simulink model "DynTaskCon"  (Simulink 7.6)
settings: Solver=ode45  StartTime=0.0  StopTime=10.0  RelTol=1e-3
InitFcn:
  | eval('Config')
values from neighbouring files (symbols this model uses):
  a2 = 0    [Config.m]    (also in CtrPlatformCfg.m)
  a3 = 0    [Config.m]    (also in CtrPlatformCfg.m)
  a4 = 0    [Config.m]    (also in CtrPlatformCfg.m)
  a5 = 90    [Config.m]    (also in CtrPlatformCfg.m)
  a6 = 0    [Config.m]    (also in CtrPlatformCfg.m)
  Cen = Cen(:)'    [Config.m]    (also in CtrPlatformCfg.m; DynEulerTest.m = Cen'; EfDynCAD.m = [cen1,cen2,cen3,cen4,cen5,cen6]')
  freq = tvel/radius    (= 1)    [Config.m]    (also in CtrPlatformCfg.m)
  Ie1 = in1(:)'    [Config.m]    (also in CtrPlatformCfg.m; DynEulerTest.m = in1(:); EfDynCAD.m = in1(:))
  Ie2 = in2(:)'    [Config.m]    (also in CtrPlatformCfg.m; DynEulerTest.m = in2(:); EfDynCAD.m = in2(:))
  Ie3 = in3(:)'    [Config.m]    (also in CtrPlatformCfg.m; DynEulerTest.m = in3(:); EfDynCAD.m = in3(:))
  Ie4 = in4(:)'    [Config.m]    (also in CtrPlatformCfg.m; DynEulerTest.m = in4(:); EfDynCAD.m = in4(:))
  Ie5 = in5(:)'    [Config.m]    (also in CtrPlatformCfg.m; DynEulerTest.m = in5(:); EfDynCAD.m = in5(:))
  Ie6 = in6(:)'    [Config.m]    (also in CtrPlatformCfg.m; DynEulerTest.m = in6(:); EfDynCAD.m = in6(:))
  init_Endx = gd_init(1,4)    [Config.m]    (also in CtrPlatformCfg.m)
  init_Endy = gd_init(2,4)    [Config.m]    (also in CtrPlatformCfg.m)
  init_Endz = gd_init(3,4)    [Config.m]    (also in CtrPlatformCfg.m)
  init_Rot = gd_init(1:3,1:3)    [Config.m]    (also in CtrPlatformCfg.m)
  L = [l1 l2 l3 l4 l5 l6 l7 l8 l9]    [Config.m]    (also in CtrPlatformCfg.m)
  Ma = [ma1 ma2 ma3 ma4 ma5 ma6]    [Config.m]    (also in CtrPlatformCfg.m; DynEulerTest.m = [ma1; ma2; ma3; ma4; ma5; ma6]; EfDynCAD.m = [ma1 ma2 ma3 ma4 ma5 ma6]')
  tvel = 120    [Config.m]    (also in CtrPlatformCfg.m)
undefined symbols (not defined in the file or in its folder): a1
libraries: mblibv1 x35, simulink x9
(part 1 of 2)
settings Model: Creator=DAI Dan  LastModifiedBy=DAI Dan
settings SimMechanicsCC: VisOnUpdateDiagram=on  VisDuringSimulation=on

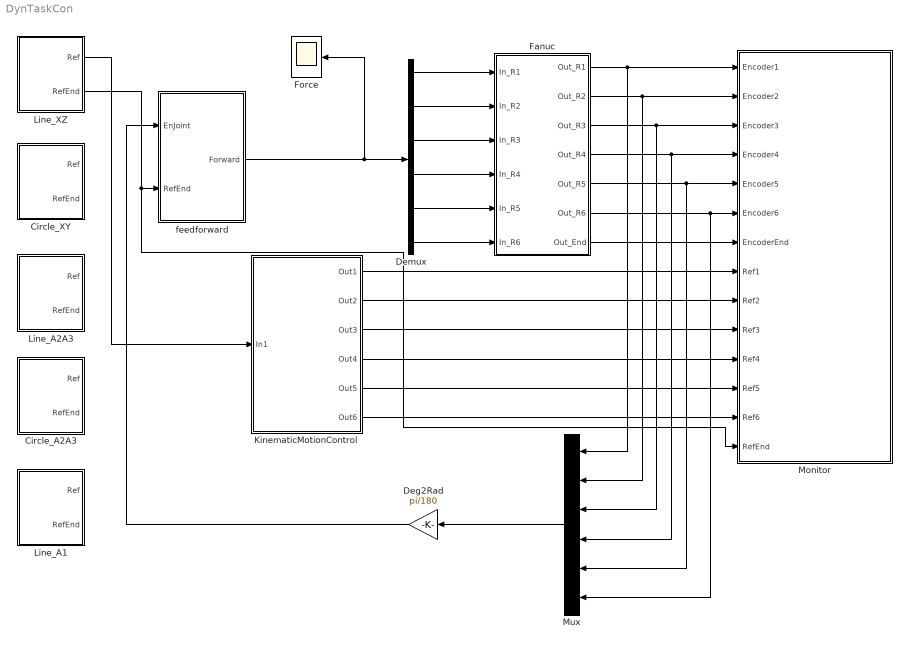
== system DynTaskCon ==
  Circle_A2A3 : Subsystem
  Circle_XY : Subsystem
  Deg2Rad : Gain  Gain=pi/180
  Demux : Demux  Outputs=6
  Fanuc : Subsystem
  Force : Scope
      settings: TimeRange=10  SaveName=ScopeData27
  KinematicMotionControl : Subsystem
  Line_A1 : Subsystem
  Line_A2A3 : Subsystem
  Line_XZ : Subsystem
  Monitor : Subsystem
  Mux : Mux  Inputs=6
  feedforward : Subsystem
  wires:
  Fanuc/1(Out_R1) -> Monitor/1(Encoder1), Mux/1
  Fanuc/2(Out_R2) -> Monitor/2(Encoder2), Mux/2
  Fanuc/3(Out_R3) -> Monitor/3(Encoder3), Mux/3
  Fanuc/4(Out_R4) -> Monitor/4(Encoder4), Mux/4
  Fanuc/5(Out_R5) -> Monitor/5(Encoder5), Mux/5
  Fanuc/6(Out_R6) -> Monitor/6(Encoder6), Mux/6
  Fanuc/7(Out_End) -> Monitor/7(EncoderEnd)
  KinematicMotionControl/1(Out1) -> Monitor/8(Ref1)
  KinematicMotionControl/2(Out2) -> Monitor/9(Ref2)
  KinematicMotionControl/3(Out3) -> Monitor/10(Ref3)
  KinematicMotionControl/4(Out4) -> Monitor/11(Ref4)
  KinematicMotionControl/5(Out5) -> Monitor/12(Ref5)
  KinematicMotionControl/6(Out6) -> Monitor/13(Ref6)
  Demux/1 -> Fanuc/1(In_R1)
  Demux/2 -> Fanuc/2(In_R2)
  Demux/3 -> Fanuc/3(In_R3)
  Demux/4 -> Fanuc/4(In_R4)
  Demux/5 -> Fanuc/5(In_R5)
  Demux/6 -> Fanuc/6(In_R6)
  Mux/1 -> Deg2Rad/1
  feedforward/1(Forward) -> Force/1, Demux/1
  Deg2Rad/1 -> feedforward/1(EnJoint)
  Line_XZ/1(Ref) -> KinematicMotionControl/1(In1)
  Line_XZ/2(RefEnd) -> Monitor/14(RefEnd), feedforward/2(RefEnd)

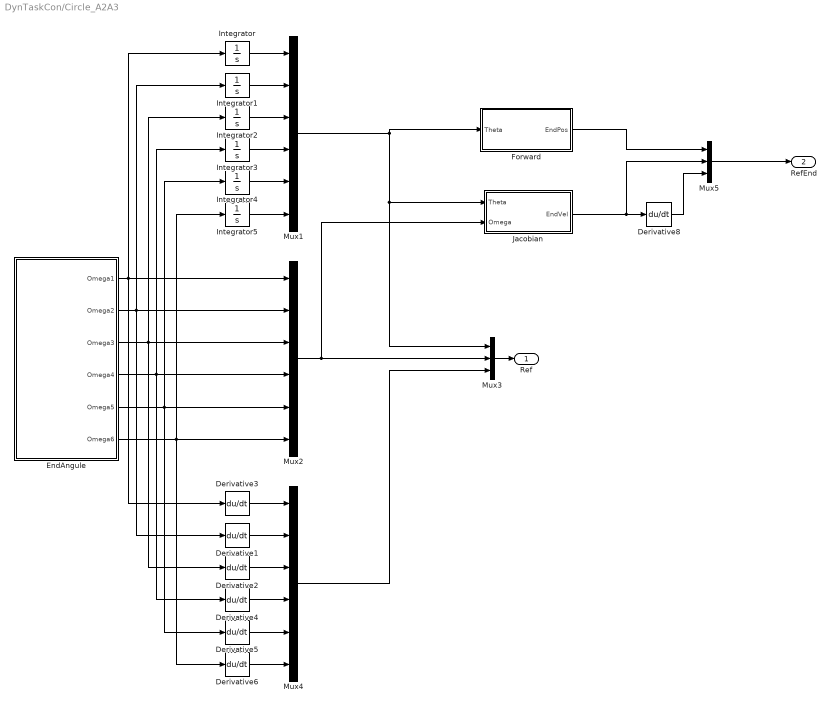
== system DynTaskCon/Circle_A2A3 ==
  Derivative{1..6,8} (7 alike) : Derivative
  EndAngule : Subsystem
  Forward : Stateflow chart  TreatAsAtomicUnit=on
  Integrator : Integrator  InitialCondition=a1/180*pi
  Integrator1 : Integrator  InitialCondition=a2/180*pi
  Integrator2 : Integrator  InitialCondition=a3/180*pi
  Integrator3 : Integrator  InitialCondition=a4/180*pi
  Integrator4 : Integrator  InitialCondition=a5/180*pi
  Integrator5 : Integrator  InitialCondition=a6/180*pi
  Jacobian : Stateflow chart  TreatAsAtomicUnit=on
  Mux1 : Mux  Inputs=6
  Mux2 : Mux  Inputs=6
  Mux3 : Mux  Inputs=3
  Mux4 : Mux  Inputs=6
  Mux5 : Mux  Inputs=3
  Ref : Outport
  RefEnd : Outport  Port=2
  wires:
  Mux3/1 -> Ref/1
  EndAngule/1(Omega1) -> Integrator/1, Mux2/1, Derivative3/1
  EndAngule/2(Omega2) -> Integrator1/1, Mux2/2, Derivative1/1
  EndAngule/3(Omega3) -> Integrator2/1, Mux2/3, Derivative2/1
  EndAngule/4(Omega4) -> Integrator3/1, Mux2/4, Derivative4/1
  EndAngule/5(Omega5) -> Integrator4/1, Mux2/5, Derivative5/1
  EndAngule/6(Omega6) -> Integrator5/1, Mux2/6, Derivative6/1
  Integrator/1 -> Mux1/1
  Integrator1/1 -> Mux1/2
  Integrator2/1 -> Mux1/3
  Integrator3/1 -> Mux1/4
  Integrator4/1 -> Mux1/5
  Integrator5/1 -> Mux1/6
  Derivative3/1 -> Mux4/1
  Derivative1/1 -> Mux4/2
  Derivative2/1 -> Mux4/3
  Derivative4/1 -> Mux4/4
  Derivative5/1 -> Mux4/5
  Derivative6/1 -> Mux4/6
  Mux2/1 -> Mux3/2, Jacobian/2(Omega)
  Mux1/1 -> Forward/1(Theta), Mux3/1, Jacobian/1(Theta)
  Mux4/1 -> Mux3/3
  Mux5/1 -> RefEnd/1
  Forward/1(EndPos) -> Mux5/1
  Jacobian/1(EndVel) -> Mux5/2, Derivative8/1
  Derivative8/1 -> Mux5/3

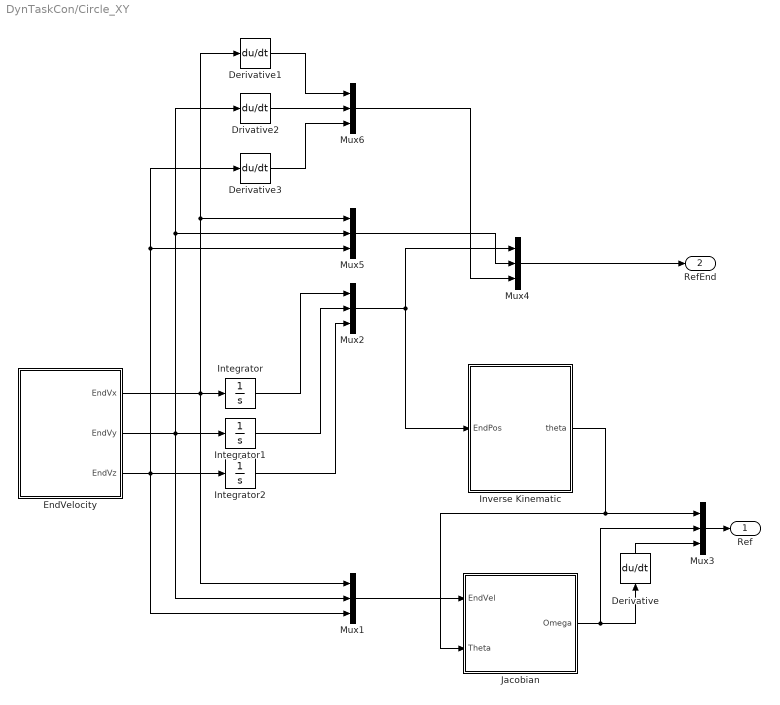
== system DynTaskCon/Circle_XY ==
  Derivative : Derivative
  Derivative1 : Derivative
  Derivative3 : Derivative
  Drivative2 : Derivative
  EndVelocity : Subsystem
  Integrator : Integrator  InitialCondition=init_Endx
  Integrator1 : Integrator  InitialCondition=init_Endy
  Integrator2 : Integrator  InitialCondition=init_Endz
  Inverse Kinematic : Stateflow chart  TreatAsAtomicUnit=on
  Jacobian : Stateflow chart  TreatAsAtomicUnit=on
  Mux{1..6} (6 alike) : Mux  Inputs=3
  Ref : Outport
  RefEnd : Outport  Port=2
  wires:
  Integrator/1 -> Mux2/1
  Integrator1/1 -> Mux2/2
  EndVelocity/1(EndVx) -> Integrator/1, Mux1/1, Mux5/1, Derivative1/1
  EndVelocity/2(EndVy) -> Integrator1/1, Mux1/2, Mux5/2, Drivative2/1
  EndVelocity/3(EndVz) -> Integrator2/1, Mux1/3, Mux5/3, Derivative3/1
  Integrator2/1 -> Mux2/3
  Mux2/1 -> Mux4/1, Inverse Kinematic/1(EndPos)
  Mux1/1 -> Jacobian/1(EndVel)
  Jacobian/1(Omega) -> Mux3/2, Derivative/1
  Mux3/1 -> Ref/1
  Derivative/1 -> Mux3/3
  Inverse Kinematic/1(theta) -> Mux3/1, Jacobian/2(Theta)
  Mux5/1 -> Mux4/2
  Mux4/1 -> RefEnd/1
  Derivative1/1 -> Mux6/1
  Drivative2/1 -> Mux6/2
  Derivative3/1 -> Mux6/3
  Mux6/1 -> Mux4/3

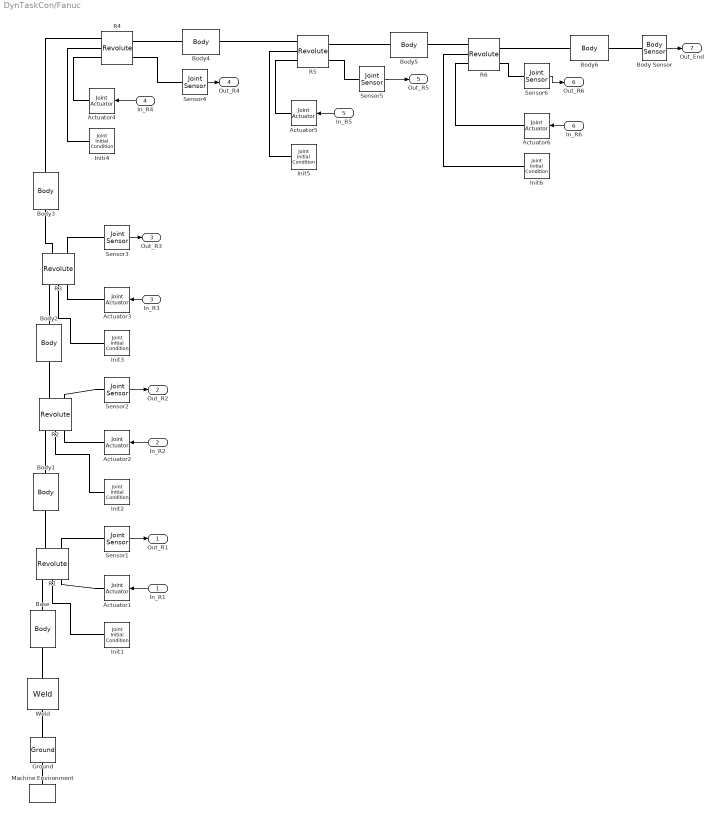
== system DynTaskCon/Fanuc ==
  In_R1 : Inport
  In_R2 : Inport  Port=2
  In_R3 : Inport  Port=3
  In_R4 : Inport  Port=4
  In_R5 : Inport  Port=5
  In_R6 : Inport  Port=6
  Actuator{1..6} (6 alike) : mblibv1/Sensors &  Actuators/Joint Actuator  DialogController=MECH.DynMechDlgSource  SystemSampleTime=-1  UpdateFromCAD=off  PhysicalDomain=Mechanical  PortType=blob  ActuationStyle=Force  AngleUnits=rad  ArcVelocityUnits=rad/s  ArcAccelerationUnits=rad/s^2  CoordPositionUnits=m  VelocityUnits=m/s  AccelerationUnits=m/s^2  ForceUnits=N  TorqueUnits=N*m  ActiveIO=on  Width=1  DialogClass=MechanicalActuatorBlock  Primitive=R1  ReferenceFrame=Absolute (World)
  Base : mblibv1/Bodies/Body  DialogController=MECH.DynMechDlgSource  PhysicalDomain=mechanical  SubClassName=Unknown  LeftPortType=workingframe  RightPortType=workingframe  LConnTagsString=CS1  RConnTagsString=CS2  UpdateFromCAD=on  DialogClass=MechanicalBodyBlock  Mass=133.95  MassUnits=kg  InertiaUnits=kg*m^2  Inertia=[3.0977 0.0155 -0.0939;0.0155 3.3580 0.0061;-0.0939 0.0061 5.1969]  Shape=Cylinder  ShapeDims=[1 1]  ShapeUnits=m  ShapeUse=false  Density=1  DensityUnits=kg/m^3  DensityUse=false  GraphicsMode=GFXFILE  GraphicsFileName=M-710iC50 M-710iC70 - M-710iC50 M-710iC70 base-1.STL  BodyColorSelMode=COLORPALETTE  BodyColor=[0.25098 0.25098 0.25098]  AttachedToCS=CS1  CG=Right$CG$[-0.0437 -0.0026 0.1059]$WORLD$WORLD$m$[1 0 0;0 1 0;0 0 1]$3x3 Transform$rad$WORLD$false$none  WorkingFrames=Left$CS1$[0 0 0]$WORLD$WORLD$m$[1 0 0;0 1 0;0 0 1]$3x3 Transform$rad$WORLD$true$none#Right$CS2$[0 0 0.266]$WORLD$WORLD$m$[1 0 0;0 1 0;0 0 1]$3x3 Transform$rad$WORLD$true$none  CGPos=[-0.0437 -0.0026 0.1059]  CGRot=[1 0 0;0 1 0;0 0 1]  CS0Pos=[]  CS0Rot=[]  CS1Pos=[0 0 0]  CS1Rot=[1 0 0;0 1 0;0 0 1]  CS2Pos=[0 0 0.266]  CS2Rot=[1 0 0;0 1 0;0 0 1]  CS3Pos=[]  CS3Rot=[]  CS4Pos=[]  CS4Rot=[]  CS5Pos=[]  CS5Rot=[]  CS6Pos=[]  CS6Rot=[]  CS7Pos=[]  CS7Rot=[]  CS8Pos=[]  CS8Rot=[]  CS9Pos=[]  CS9Rot=[]  CS10Pos=[]  CS10Rot=[]  CS11Pos=[]  CS11Rot=[]  CS12Pos=[]  CS12Rot=[]  CS13Pos=[]  CS13Rot=[]  CS14Pos=[]  CS14Rot=[]  CS15Pos=[]  CS15Rot=[]  CS16Pos=[]  CS16Rot=[]  CS17Pos=[]  CS17Rot=[]  CS18Pos=[]  CS18Rot=[]  CS19Pos=[]  CS19Rot=[]  CS20Pos=[]  CS20Rot=[]
  Body Sensor : mblibv1/Sensors &  Actuators/Body Sensor  DialogController=MECH.DynMechDlgSource  SystemSampleTime=-1  UpdateFromCAD=off  PhysicalDomain=Mechanical  PortType=blob  Muxed=on  Pose=off  Angle=on  AngleUnits=deg  ArcVelocity=off  ArcVelocityUnits=deg/s  ArcAcceleration=off  ArcAccelerationUnits=deg/s^2  CoordPosition=on  CoordPositionUnits=mm  Velocity=on  VelocityUnits=mm/s  Acceleration=on  AccelerationUnits=mm/s^2  Quaternion=on  QuaternionDT=off  QuaternionDDT=off  QuaternionUnits=off  OutputVector=[1]  ActiveIO=on  Width=9  DialogClass=MechanicalSensorBlock  ReferenceFrame=Absolute (World)
  Body1 : mblibv1/Bodies/Body  DialogController=MECH.DynMechDlgSource  PhysicalDomain=mechanical  SubClassName=Unknown  LeftPortType=workingframe  RightPortType=workingframe  LConnTagsString=CS2  RConnTagsString=CS3  UpdateFromCAD=on  DialogClass=MechanicalBodyBlock  Mass=170.31  MassUnits=kg  InertiaUnits=kg*m^2  Inertia=[5.2954 -0.2565 -0.6366;-0.2565 4.7000 0.2830;-0.6366 0.2829 5.8635]  Shape=Cylinder  ShapeDims=[1 1]  ShapeUnits=m  ShapeUse=false  Density=1  DensityUnits=kg/m^3  DensityUse=false  GraphicsMode=GFXFILE  GraphicsFileName=M-710iC50 M-710iC70 - M-710iC50 M-710iC70 axis1-1.STL  BodyColorSelMode=COLORPALETTE  BodyColor=[0.86667 0.86667 0.8902]  AttachedToCS=CS1  CG=Right$CG$[0.0407 -0.0528 0.4702]$WORLD$WORLD$m$[1 0 0;0 1 0;0 0 1]$3x3 Transform$rad$WORLD$false$none  WorkingFrames=Right$CS1$[0 0 0]$WORLD$WORLD$m$[1 0 0;0 1 0;0 0 1]$3x3 Transform$rad$WORLD$false$none#Left$CS2$[0 0 0.266]$WORLD$WORLD$m$[1 0 0;0 1 0;0 0 1]$3x3 Transform$rad$WORLD$true$none#Right$CS3$[0.15 0.062 0.566]$WORLD$WORLD$m$[1 0 0;0 1 0;0 0 1]$3x3 Transform$rad$WORLD$true$none  CGPos=[0.0407 -0.0528 0.4702]  CGRot=[1 0 0;0 1 0;0 0 1]  CS0Pos=[]  CS0Rot=[]  CS1Pos=[0 0 0]  CS1Rot=[1 0 0;0 1 0;0 0 1]  CS2Pos=[0 0 0.266]  CS2Rot=[1 0 0;0 1 0;0 0 1]  CS3Pos=[0.15 0.062 0.566]  CS3Rot=[1 0 0;0 1 0;0 0 1]  CS4Pos=[]  CS4Rot=[]  CS5Pos=[]  CS5Rot=[]  CS6Pos=[]  CS6Rot=[]  CS7Pos=[]  CS7Rot=[]  CS8Pos=[]  CS8Rot=[]  CS9Pos=[]  CS9Rot=[]  CS10Pos=[]  CS10Rot=[]  CS11Pos=[]  CS11Rot=[]  CS12Pos=[]  CS12Rot=[]  CS13Pos=[]  CS13Rot=[]  CS14Pos=[]  CS14Rot=[]  CS15Pos=[]  CS15Rot=[]  CS16Pos=[]  CS16Rot=[]  CS17Pos=[]  CS17Rot=[]  CS18Pos=[]  CS18Rot=[]  CS19Pos=[]  CS19Rot=[]  CS20Pos=[]  CS20Rot=[]
  Body2 : mblibv1/Bodies/Body  DialogController=MECH.DynMechDlgSource  PhysicalDomain=mechanical  SubClassName=Unknown  LeftPortType=workingframe  RightPortType=workingframe  LConnTagsString=CS2  RConnTagsString=CS3  UpdateFromCAD=on  DialogClass=MechanicalBodyBlock  Mass=63.74  MassUnits=kg  InertiaUnits=kg*m^2  Inertia=[5.8840 0.0072 0.0135;0.0072 6.0178 -0.1907;0.0135 -0.1907 0.3374]  Shape=Cylinder  ShapeDims=[1 1]  ShapeUnits=m  ShapeUse=false  Density=1  DensityUnits=kg/m^3  DensityUse=false  GraphicsMode=GFXFILE  GraphicsFileName=M-710iC50 M-710iC70 - M-710iC50 M-710iC70 axis2-1.STL  BodyColorSelMode=COLORPALETTE  BodyColor=[1 1 0]  AttachedToCS=CS1  CG=Right$CG$[0.1510 0.1746 0.9687]$WORLD$WORLD$m$[1 0 0;0 1 0;0 0 1]$3x3 Transform$rad$WORLD$false$none  WorkingFrames=Right$CS1$[0 0 0]$WORLD$WORLD$m$[1 0 0;0 1 0;0 0 1]$3x3 Transform$rad$WORLD$false$none#Left$CS2$[0.15 0.062 0.566]$WORLD$WORLD$m$[1 0 0;0 1 0;0 0 1]$3x3 Transform$rad$WORLD$true$none#Right$CS3$[0.15 0.227 1.436]$WORLD$WORLD$m$[1 0 0;0 1 0;0 0 1]$3x3 Transform$rad$WORLD$true$none  CGPos=[0.1510 0.1746 0.9687]  CGRot=[1 0 0;0 1 0;0 0 1]  CS0Pos=[]  CS0Rot=[]  CS1Pos=[0 0 0]  CS1Rot=[1 0 0;0 1 0;0 0 1]  CS2Pos=[0.15 0.062 0.566]  CS2Rot=[1 0 0;0 1 0;0 0 1]  CS3Pos=[0.15 0.227 1.436]  CS3Rot=[1 0 0;0 1 0;0 0 1]  CS4Pos=[]  CS4Rot=[]  CS5Pos=[]  CS5Rot=[]  CS6Pos=[]  CS6Rot=[]  CS7Pos=[]  CS7Rot=[]  CS8Pos=[]  CS8Rot=[]  CS9Pos=[]  CS9Rot=[]  CS10Pos=[]  CS10Rot=[]  CS11Pos=[]  CS11Rot=[]  CS12Pos=[]  CS12Rot=[]  CS13Pos=[]  CS13Rot=[]  CS14Pos=[]  CS14Rot=[]  CS15Pos=[]  CS15Rot=[]  CS16Pos=[]  CS16Rot=[]  CS17Pos=[]  CS17Rot=[]  CS18Pos=[]  CS18Rot=[]  CS19Pos=[]  CS19Rot=[]  CS20Pos=[]  CS20Rot=[]
  Body3 : mblibv1/Bodies/Body  DialogController=MECH.DynMechDlgSource  PhysicalDomain=mechanical  SubClassName=Unknown  LeftPortType=workingframe  RightPortType=workingframe  LConnTagsString=CS2  RConnTagsString=CS3  UpdateFromCAD=on  DialogClass=MechanicalBodyBlock  Mass=98.98  MassUnits=kg  InertiaUnits=kg*m^2  Inertia=[1.8201 -0.2274 -0.3112;-0.2274 2.2537 -0.1441;-0.3112 -0.1441 1.9485]  Shape=Cylinder  ShapeDims=[1 1]  ShapeUnits=m  ShapeUse=false  Density=1  DensityUnits=kg/m^3  DensityUse=false  GraphicsMode=GFXFILE  GraphicsFileName=M-710iC50 M-710iC70 - M-710iC50 M-710iC70 axis3-1.STL  BodyColorSelMode=COLORPALETTE  BodyColor=[1 1 0]  AttachedToCS=CS1  CG=Right$CG$[0.1568 -0.0318 1.5191]$WORLD$WORLD$m$[1 0 0;0 1 0;0 0 1]$3x3 Transform$rad$WORLD$false$none  WorkingFrames=Right$CS1$[0 0 0]$WORLD$WORLD$m$[1 0 0;0 1 0;0 0 1]$3x3 Transform$rad$WORLD$false$none#Left$CS2$[0.15 0.227 1.436]$WORLD$WORLD$m$[1 0 0;0 1 0;0 0 1]$3x3 Transform$rad$WORLD$true$none#Right$CS3$[0.510 0 1.606]$WORLD$WORLD$m$[1 0 0;0 1 0;0 0 1]$3x3 Transform$rad$WORLD$true$none  CGPos=[0.1568 -0.0318 1.5191]  CGRot=[1 0 0;0 1 0;0 0 1]  CS0Pos=[]  CS0Rot=[]  CS1Pos=[0 0 0]  CS1Rot=[1 0 0;0 1 0;0 0 1]  CS2Pos=[0.15 0.227 1.436]  CS2Rot=[1 0 0;0 1 0;0 0 1]  CS3Pos=[0.510 0 1.606]  CS3Rot=[1 0 0;0 1 0;0 0 1]  CS4Pos=[]  CS4Rot=[]  CS5Pos=[]  CS5Rot=[]  CS6Pos=[]  CS6Rot=[]  CS7Pos=[]  CS7Rot=[]  CS8Pos=[]  CS8Rot=[]  CS9Pos=[]  CS9Rot=[]  CS10Pos=[]  CS10Rot=[]  CS11Pos=[]  CS11Rot=[]  CS12Pos=[]  CS12Rot=[]  CS13Pos=[]  CS13Rot=[]  CS14Pos=[]  CS14Rot=[]  CS15Pos=[]  CS15Rot=[]  CS16Pos=[]  CS16Rot=[]  CS17Pos=[]  CS17Rot=[]  CS18Pos=[]  CS18Rot=[]  CS19Pos=[]  CS19Rot=[]  CS20Pos=[]  CS20Rot=[]
  Body4 : mblibv1/Bodies/Body  DialogController=MECH.DynMechDlgSource  PhysicalDomain=mechanical  SubClassName=Unknown  LeftPortType=workingframe  RightPortType=workingframe  LConnTagsString=CS2  RConnTagsString=CS3  UpdateFromCAD=on  DialogClass=MechanicalBodyBlock  Mass=24.46  MassUnits=kg  InertiaUnits=kg*m^2  Inertia=[0.0607 -0.0922 0;-0.0922 1.4493 0;0 0,1.4620]  Shape=Cylinder  ShapeDims=[1 1]  ShapeUnits=m  ShapeUse=false  Density=1  DensityUnits=kg/m^3  DensityUse=false  GraphicsMode=GFXFILE  GraphicsFileName=M-710iC50 M-710iC70 - M-710iC50 M-710iC70 axis4-1.STL  BodyColorSelMode=COLORPALETTE  BodyColor=[1 1 0]  AttachedToCS=CS1  CG=Right$CG$[0.8245 -0.0110 1.606]$WORLD$WORLD$m$[1 0 0;0 0 1;0 -1 0]$3x3 Transform$rad$WORLD$false$none  WorkingFrames=Right$CS1$[0.4525 0 1.606]$WORLD$WORLD$m$[1 0 0;0 0 1;0 -1 0]$3x3 Transform$rad$WORLD$false$none#Left$CS2$[0.510 0 1.606]$WORLD$WORLD$m$[1 0 0;0 1 0;0 0 1]$3x3 Transform$rad$WORLD$true$none#Right$CS3$[1.166 -0.113 1.606]$WORLD$WORLD$m$[1 0 0;0 1 0;0 0 1]$3x3 Transform$rad$WORLD$true$none  CGPos=[0.8245 -0.0110 1.606]  CGRot=[1 0 0;0 0 1;0 -1 0]  CS0Pos=[]  CS0Rot=[]  CS1Pos=[0.4525 0 1.606]  CS1Rot=[1 0 0;0 0 1;0 -1 0]  CS2Pos=[0.510 0 1.606]  CS2Rot=[1 0 0;0 1 0;0 0 1]  CS3Pos=[1.166 -0.113 1.606]  CS3Rot=[1 0 0;0 1 0;0 0 1]  CS4Pos=[]  CS4Rot=[]  CS5Pos=[]  CS5Rot=[]  CS6Pos=[]  CS6Rot=[]  CS7Pos=[]  CS7Rot=[]  CS8Pos=[]  CS8Rot=[]  CS9Pos=[]  CS9Rot=[]  CS10Pos=[]  CS10Rot=[]  CS11Pos=[]  CS11Rot=[]  CS12Pos=[]  CS12Rot=[]  CS13Pos=[]  CS13Rot=[]  CS14Pos=[]  CS14Rot=[]  CS15Pos=[]  CS15Rot=[]  CS16Pos=[]  CS16Rot=[]  CS17Pos=[]  CS17Rot=[]  CS18Pos=[]  CS18Rot=[]  CS19Pos=[]  CS19Rot=[]  CS20Pos=[]  CS20Rot=[]
  Body5 : mblibv1/Bodies/Body  DialogController=MECH.DynMechDlgSource  PhysicalDomain=mechanical  SubClassName=Unknown  LeftPortType=workingframe  RightPortType=workingframe  LConnTagsString=CS2  RConnTagsString=CS3  UpdateFromCAD=on  DialogClass=MechanicalBodyBlock  Mass=5.24  MassUnits=kg  InertiaUnits=kg*m^2  Inertia=[0.0191 0.0032 0;0.0032 0.0228 0;0 0 0.0291]  Shape=Cylinder  ShapeDims=[1 1]  ShapeUnits=m  ShapeUse=false  Density=1  DensityUnits=kg/m^3  DensityUse=false  GraphicsMode=GFXFILE  GraphicsFileName=M-710iC50 M-710iC70 - M-710iC50 M-710iC70 axis5-1.STL  BodyColorSelMode=COLORPALETTE  BodyColor=[1 1 0]  AttachedToCS=CS1  CG=Right$CG$[1.2407 0.0180 1.606]$WORLD$WORLD$m$[1 0 0;0 1 0;0 0 1]$3x3 Transform$rad$WORLD$false$none  WorkingFrames=Right$CS1$[0 0 0]$WORLD$WORLD$m$[1 0 0;0 1 0;0 0 1]$3x3 Transform$rad$WORLD$false$none#Left$CS2$[1.166 -0.113 1.606]$WORLD$WORLD$m$[1 0 0;0 1 0;0 0 1]$3x3 Transform$rad$WORLD$true$none#Right$CS3$[1.320 0 1.606]$WORLD$WORLD$m$[1 0 0;0 1 0;0 0 1]$3x3 Transform$rad$WORLD$true$none  CGPos=[1.2407 0.0180 1.606]  CGRot=[1 0 0;0 1 0;0 0 1]  CS0Pos=[]  CS0Rot=[]  CS1Pos=[0 0 0]  CS1Rot=[1 0 0;0 1 0;0 0 1]  CS2Pos=[1.166 -0.113 1.606]  CS2Rot=[1 0 0;0 1 0;0 0 1]  CS3Pos=[1.320 0 1.606]  CS3Rot=[1 0 0;0 1 0;0 0 1]  CS4Pos=[]  CS4Rot=[]  CS5Pos=[]  CS5Rot=[]  CS6Pos=[]  CS6Rot=[]  CS7Pos=[]  CS7Rot=[]  CS8Pos=[]  CS8Rot=[]  CS9Pos=[]  CS9Rot=[]  CS10Pos=[]  CS10Rot=[]  CS11Pos=[]  CS11Rot=[]  CS12Pos=[]  CS12Rot=[]  CS13Pos=[]  CS13Rot=[]  CS14Pos=[]  CS14Rot=[]  CS15Pos=[]  CS15Rot=[]  CS16Pos=[]  CS16Rot=[]  CS17Pos=[]  CS17Rot=[]  CS18Pos=[]  CS18Rot=[]  CS19Pos=[]  CS19Rot=[]  CS20Pos=[]  CS20Rot=[]
  Body6 : mblibv1/Bodies/Body  DialogController=MECH.DynMechDlgSource  PhysicalDomain=mechanical  SubClassName=Unknown  LeftPortType=workingframe  RightPortType=workingframe  LConnTagsString=CS2  RConnTagsString=CS3  UpdateFromCAD=on  DialogClass=MechanicalBodyBlock  Mass=0.6  MassUnits=kg  InertiaUnits=kg*m^2  Inertia=[0.0012 0 0;0 0.0007 0;0 0 0.0007]  Shape=Cylinder  ShapeDims=[1 1]  ShapeUnits=m  ShapeUse=false  Density=1  DensityUnits=kg/m^3  DensityUse=false  GraphicsMode=GFXFILE  GraphicsFileName=M-710iC50 M-710iC70 - M-710iC50 M-710iC70 axis6-1.STL  BodyColorSelMode=COLORPALETTE  BodyColor=[0.75294 0.75294 0.75294]  AttachedToCS=CS1  CG=Right$CG$[1.330 0 1.606]$WORLD$WORLD$m$[1 0 0;0 1 0;0 0 1]$3x3 Transform$rad$WORLD$false$none  WorkingFrames=Right$CS1$[1.34 0 1.606]$WORLD$WORLD$m$[0 0 1;0 -1 0;1 0 0]$3x3 Transform$rad$WORLD$false$none#Left$CS2$[1.320 0 1.606]$WORLD$WORLD$m$[1 0 0;0 1 0;0 0 1]$3x3 Transform$rad$WORLD$true$none#Right$CS3$[1.34 0 1.606]$WORLD$WORLD$m$[1 0 0;0 1 0;0 0 1]$3x3 Transform$rad$WORLD$true$none  CGPos=[1.330 0 1.606]  CGRot=[1 0 0;0 1 0;0 0 1]  CS0Pos=[]  CS0Rot=[]  CS1Pos=[1.34 0 1.606]  CS1Rot=[0 0 1;0 -1 0;1 0 0]  CS2Pos=[1.320 0 1.606]  CS2Rot=[1 0 0;0 1 0;0 0 1]  CS3Pos=[1.34 0 1.606]  CS3Rot=[1 0 0;0 1 0;0 0 1]  CS4Pos=[]  CS4Rot=[]  CS5Pos=[]  CS5Rot=[]  CS6Pos=[]  CS6Rot=[]  CS7Pos=[]  CS7Rot=[]  CS8Pos=[]  CS8Rot=[]  CS9Pos=[]  CS9Rot=[]  CS10Pos=[]  CS10Rot=[]  CS11Pos=[]  CS11Rot=[]  CS12Pos=[]  CS12Rot=[]  CS13Pos=[]  CS13Rot=[]  CS14Pos=[]  CS14Rot=[]  CS15Pos=[]  CS15Rot=[]  CS16Pos=[]  CS16Rot=[]  CS17Pos=[]  CS17Rot=[]  CS18Pos=[]  CS18Rot=[]  CS19Pos=[]  CS19Rot=[]  CS20Pos=[]  CS20Rot=[]
  Ground : mblibv1/Bodies/Ground  DialogController=MECH.DynMechDlgSource  SystemSampleTime=-1  UpdateFromCAD=on  LeftPortType=env  RightPortType=workingframe  PhysicalDomain=Mechanical  DialogClass=GroundBlock  CoordPosition=[0 0 0]  CoordPositionUnits=m  StateVectorMgrId=0  MachineId=[1 0]  ShowEnvPort=on
  Init1 : mblibv1/Sensors &  Actuators/Joint Initial Condition  DialogController=MECH.DynMechDlgSource  SystemSampleTime=-1  UpdateFromCAD=off  LeftPortType=blob  RightPortType=blob  PhysicalDomain=mechanical  DialogClass=InitialConditionBlock  InitialConditions=P1$false$0$m$deg$0$m/s$deg/s#P2$false$0$m$deg$0$m/s$deg/s#P3$false$0$m$deg$0$m/s$deg/s#R1$true$a1$m$deg$0$m/s$deg/s#R2$false$0$m$deg$0$m/s$deg/s#R3$false$0$m$deg$0$m/s$deg/s#S$false$0$m$deg$0$m/s$deg/s  P1PIC=0  P1VIC=0  P2PIC=0  P2VIC=0  P3PIC=0  P3VIC=0  R1PIC=a1  R1VIC=0  R2PIC=0  R2VIC=0  R3PIC=0  R3VIC=0  SPIC=0  SVIC=0
  Init2 : mblibv1/Sensors &  Actuators/Joint Initial Condition  DialogController=MECH.DynMechDlgSource  SystemSampleTime=-1  UpdateFromCAD=off  LeftPortType=blob  RightPortType=blob  PhysicalDomain=mechanical  DialogClass=InitialConditionBlock  InitialConditions=P1$false$0$m$deg$0$m/s$deg/s#P2$false$0$m$deg$0$m/s$deg/s#P3$false$0$m$deg$0$m/s$deg/s#R1$true$a2$m$deg$0$m/s$deg/s#R2$false$0$m$deg$0$m/s$deg/s#R3$false$0$m$deg$0$m/s$deg/s#S$false$0$m$deg$0$m/s$deg/s  P1PIC=0  P1VIC=0  P2PIC=0  P2VIC=0  P3PIC=0  P3VIC=0  R1PIC=a2  R1VIC=0  R2PIC=0  R2VIC=0  R3PIC=0  R3VIC=0  SPIC=0  SVIC=0
  Init3 : mblibv1/Sensors &  Actuators/Joint Initial Condition  DialogController=MECH.DynMechDlgSource  SystemSampleTime=-1  UpdateFromCAD=off  LeftPortType=blob  RightPortType=blob  PhysicalDomain=mechanical  DialogClass=InitialConditionBlock  InitialConditions=P1$false$0$m$deg$0$m/s$deg/s#P2$false$0$m$deg$0$m/s$deg/s#P3$false$0$m$deg$0$m/s$deg/s#R1$true$a3$m$deg$0$m/s$deg/s#R2$false$0$m$deg$0$m/s$deg/s#R3$false$0$m$deg$0$m/s$deg/s#S$false$0$m$deg$0$m/s$deg/s  P1PIC=0  P1VIC=0  P2PIC=0  P2VIC=0  P3PIC=0  P3VIC=0  R1PIC=a3  R1VIC=0  R2PIC=0  R2VIC=0  R3PIC=0  R3VIC=0  SPIC=0  SVIC=0
  Init5 : mblibv1/Sensors &  Actuators/Joint Initial Condition  DialogController=MECH.DynMechDlgSource  SystemSampleTime=-1  UpdateFromCAD=off  LeftPortType=blob  RightPortType=blob  PhysicalDomain=mechanical  DialogClass=InitialConditionBlock  InitialConditions=P1$false$0$m$deg$0$m/s$deg/s#P2$false$0$m$deg$0$m/s$deg/s#P3$false$0$m$deg$0$m/s$deg/s#R1$true$a5$m$deg$0$m/s$deg/s#R2$false$0$m$deg$0$m/s$deg/s#R3$false$0$m$deg$0$m/s$deg/s#S$false$0$m$deg$0$m/s$deg/s  P1PIC=0  P1VIC=0  P2PIC=0  P2VIC=0  P3PIC=0  P3VIC=0  R1PIC=a5  R1VIC=0  R2PIC=0  R2VIC=0  R3PIC=0  R3VIC=0  SPIC=0  SVIC=0
  Init6 : mblibv1/Sensors &  Actuators/Joint Initial Condition  DialogController=MECH.DynMechDlgSource  SystemSampleTime=-1  UpdateFromCAD=off  LeftPortType=blob  RightPortType=blob  PhysicalDomain=mechanical  DialogClass=InitialConditionBlock  InitialConditions=P1$false$0$m$deg$0$m/s$deg/s#P2$false$0$m$deg$0$m/s$deg/s#P3$false$0$m$deg$0$m/s$deg/s#R1$true$a6$m$deg$0$m/s$deg/s#R2$false$0$m$deg$0$m/s$deg/s#R3$false$0$m$deg$0$m/s$deg/s#S$false$0$m$deg$0$m/s$deg/s  P1PIC=0  P1VIC=0  P2PIC=0  P2VIC=0  P3PIC=0  P3VIC=0  R1PIC=a6  R1VIC=0  R2PIC=0  R2VIC=0  R3PIC=0  R3VIC=0  SPIC=0  SVIC=0
  Initi4 : mblibv1/Sensors &  Actuators/Joint Initial Condition  DialogController=MECH.DynMechDlgSource  SystemSampleTime=-1  UpdateFromCAD=off  LeftPortType=blob  RightPortType=blob  PhysicalDomain=mechanical  DialogClass=InitialConditionBlock  InitialConditions=P1$false$0$m$deg$0$m/s$deg/s#P2$false$0$m$deg$0$m/s$deg/s#P3$false$0$m$deg$0$m/s$deg/s#R1$true$a4$m$deg$0$m/s$deg/s#R2$false$0$m$deg$0$m/s$deg/s#R3$false$0$m$deg$0$m/s$deg/s#S$false$0$m$deg$0$m/s$deg/s  P1PIC=0  P1VIC=0  P2PIC=0  P2VIC=0  P3PIC=0  P3VIC=0  R1PIC=a4  R1VIC=0  R2PIC=0  R2VIC=0  R3PIC=0  R3VIC=0  SPIC=0  SVIC=0
  Machine Environment : mblibv1/Bodies/Machine Environment  DialogController=MECH.DialogSource  SystemSampleTime=-1  PortType=env  PhysicalDomain=Mechanical  DialogTemplateClass=MECH.MachineEnvironment  SyncWhenCopied=off  Gravity=[0 0 0]  GravityUnits=m/s^2  GravityAsSignal=off  Dimensionality=Auto-detect  AnalysisType=Forward dynamics  LinearAssemblyTolerance=1e-3  LinearAssemblyToleranceUnits=m  AngularAssemblyTolerance=1e-3  AngularAssemblyToleranceUnits=rad  ConstraintSolverType=Stabilizing  ConstraintRelTolerance=1e-4  ConstraintAbsTolerance=1e-4  UseRobustSingularityHandling=off  RedundancyAnalysisToleranceType=Automatically select tolerance  RedundancyAnalysisTolerance=1e-14  StatePerturbationType=Fixed  PerturbationSize=1e-5  VisualizeMachine=on  BodyVisualizationType=Use model default body geometries  BodyColorSelMode=Use model default  DefaultBodyColor=[1 0 0]
  R1 : mblibv1/Joints/Revolute  DialogController=MECH.DynMechDlgSource  PhysicalDomain=mechanical  SubClassName=Unknown  LeftPortType=blob  RightPortType=blob  LConnTagsString=__newl0|SA1|SA2  RConnTagsString=__newr0|SA1  UpdateFromCAD=on  NumSAPorts=3  CutJoint=off  MarkAsCut=off  Primitives=prismatic  PrimitiveProps=R1$World$[0,0,1]$revolute  DialogClass=JointBlock  R1Axis=[0,0,1]
  R2 : mblibv1/Joints/Revolute  DialogController=MECH.DynMechDlgSource  PhysicalDomain=mechanical  SubClassName=Unknown  LeftPortType=blob  RightPortType=blob  LConnTagsString=__newl0|SA1|SA2  RConnTagsString=__newr0|SA1  UpdateFromCAD=on  NumSAPorts=3  CutJoint=off  MarkAsCut=off  Primitives=prismatic  PrimitiveProps=R1$World$[0,1,0]$revolute  DialogClass=JointBlock  R1Axis=[0,1,0]
  R3 : mblibv1/Joints/Revolute  DialogController=MECH.DynMechDlgSource  PhysicalDomain=mechanical  SubClassName=Unknown  LeftPortType=blob  RightPortType=blob  LConnTagsString=__newl0|SA1|SA2  RConnTagsString=__newr0|SA1  UpdateFromCAD=on  NumSAPorts=3  CutJoint=off  MarkAsCut=off  Primitives=prismatic  PrimitiveProps=R1$World$[0,1,0]$revolute  DialogClass=JointBlock  R1Axis=[0,1,0]
  R4 : mblibv1/Joints/Revolute  DialogController=MECH.DynMechDlgSource  PhysicalDomain=mechanical  SubClassName=Unknown  LeftPortType=blob  RightPortType=blob  LConnTagsString=__newl0|SA1|SA2  RConnTagsString=__newr0|SA1  UpdateFromCAD=on  NumSAPorts=3  CutJoint=off  MarkAsCut=off  Primitives=prismatic  PrimitiveProps=R1$World$[1,0,0]$revolute  DialogClass=JointBlock  R1Axis=[1,0,0]
  R5 : mblibv1/Joints/Revolute  DialogController=MECH.DynMechDlgSource  PhysicalDomain=mechanical  SubClassName=Unknown  LeftPortType=blob  RightPortType=blob  LConnTagsString=__newl0|SA1|SA2  RConnTagsString=__newr0|SA1  UpdateFromCAD=on  NumSAPorts=3  CutJoint=off  MarkAsCut=off  Primitives=prismatic  PrimitiveProps=R1$World$[0,1,0]$revolute  DialogClass=JointBlock  R1Axis=[0,1,0]
  R6 : mblibv1/Joints/Revolute  DialogController=MECH.DynMechDlgSource  PhysicalDomain=mechanical  SubClassName=Unknown  LeftPortType=blob  RightPortType=blob  LConnTagsString=__newl0|SA1|SA2  RConnTagsString=__newr0|SA1  UpdateFromCAD=on  NumSAPorts=3  CutJoint=off  MarkAsCut=off  Primitives=prismatic  PrimitiveProps=R1$World$[1,0,0]$revolute  DialogClass=JointBlock  R1Axis=[1,0,0]
  Sensor1 : mblibv1/Sensors &  Actuators/Joint Sensor  DialogController=MECH.DynMechDlgSource  SystemSampleTime=-1  UpdateFromCAD=off  PhysicalDomain=Mechanical  PortType=blob  Muxed=on  Pose=off  Angle=on  AngleUnits=deg  ArcVelocity=on  ArcVelocityUnits=deg/s  ArcAcceleration=on  ArcAccelerationUnits=deg/s^2  CoordPosition=on  CoordPositionUnits=m  Velocity=off  VelocityUnits=m/s  Acceleration=off  AccelerationUnits=m/s^2  Quaternion=on  QuaternionDT=off  QuaternionDDT=off  QuaternionUnits=off  OutputVector=[1]  ActiveIO=on  Width=3  DialogClass=MechanicalSensorBlock  Primitive=R1  Force=off  ForceUnits=N  Torque=off  TorqueUnits=N*m  ReferenceFrame=Absolute (World)  ReactionSensedSide=Follower  ReactionReferenceFrame=Absolute (World)  ReactionForce=off  ReactionForceUnits=N  ReactionMoment=off  ReactionMomentUnits=N*m
  Sensor{2..6} (5 alike) : mblibv1/Sensors &  Actuators/Joint Sensor  DialogController=MECH.DynMechDlgSource  SystemSampleTime=-1  UpdateFromCAD=off  PhysicalDomain=Mechanical  PortType=blob  Muxed=on  Pose=off  Angle=on  AngleUnits=deg  ArcVelocity=on  ArcVelocityUnits=deg/s  ArcAcceleration=on  ArcAccelerationUnits=deg/s^2  CoordPosition=on  CoordPositionUnits=m  Velocity=off  VelocityUnits=m/s  Acceleration=off  AccelerationUnits=m/s^2  Quaternion=on  QuaternionDT=off  QuaternionDDT=off  QuaternionUnits=off  OutputVector=[1]  ActiveIO=on  Width=3  DialogClass=MechanicalSensorBlock  Primitive=R1  Force=off  ForceUnits=N  Torque=off  TorqueUnits=N*m  ReferenceFrame=Absolute (World)  ReactionSensedSide=Base  ReactionReferenceFrame=Absolute (World)  ReactionForce=off  ReactionForceUnits=N  ReactionMoment=off  ReactionMomentUnits=N*m
  Weld : mblibv1/Joints/Weld  DialogController=MECH.DynMechDlgSource  PhysicalDomain=mechanical  SubClassName=Unknown  LeftPortType=blob  RightPortType=blob  LConnTagsString=__newl0  RConnTagsString=__newr0  UpdateFromCAD=on  NumSAPorts=0  CutJoint=off  MarkAsCut=off  Primitives=weld  PrimitiveProps=W$WORLD$[0.57735,0.57735,0.57735]$weld  DialogClass=JointBlock  WAxis=[0.57735,0.57735,0.57735]
  Out_R1 : Outport
  Out_R2 : Outport  Port=2
  Out_R3 : Outport  Port=3
  Out_R4 : Outport  Port=4
  Out_R5 : Outport  Port=5
  Out_R6 : Outport  Port=6
  Out_End : Outport  Port=7
  wires:
  In_R1/1 -> Actuator1/1
  Sensor1/1 -> Out_R1/1
  In_R2/1 -> Actuator2/1
  Sensor2/1 -> Out_R2/1
  In_R3/1 -> Actuator3/1
  Sensor3/1 -> Out_R3/1
  Sensor4/1 -> Out_R4/1
  In_R4/1 -> Actuator4/1
  Sensor5/1 -> Out_R5/1
  In_R5/1 -> Actuator5/1
  Sensor6/1 -> Out_R6/1
  In_R6/1 -> Actuator6/1
  Body Sensor/1 -> Out_End/1
  connections:
  Body Sensor/LConn1 -- Body6/RConn1
  Sensor6/LConn1 -- R6/RConn2
  Actuator6/RConn1 -- R6/LConn3
  Weld/LConn1 -- Ground/RConn1
  Actuator3/RConn1 -- R3/LConn3
  Init3/RConn1 -- R3/LConn2
  Sensor3/LConn1 -- R3/RConn2
  Machine Environment/RConn1 -- Ground/LConn1
  R5/LConn1 -- Body4/RConn1
  R1/LConn1 -- Base/RConn1
  R6/RConn1 -- Body6/LConn1
  R5/RConn1 -- Body5/LConn1
  Body5/RConn1 -- R6/LConn1
  Body2/RConn1 -- R3/LConn1
  R2/RConn1 -- Body2/LConn1
  R2/LConn1 -- Body1/RConn1
  Weld/RConn1 -- Base/LConn1
  Actuator2/RConn1 -- R2/LConn3
  Init6/RConn1 -- R6/LConn2
  Body1/LConn1 -- R1/RConn1
  Sensor2/LConn1 -- R2/RConn2
  Init2/RConn1 -- R2/LConn2
  R1/RConn2 -- Sensor1/LConn1
  Actuator1/RConn1 -- R1/LConn3
  R1/LConn2 -- Init1/RConn1
  Sensor5/LConn1 -- R5/RConn2
  R3/RConn1 -- Body3/LConn1
  Actuator5/RConn1 -- R5/LConn3
  Init5/RConn1 -- R5/LConn2
  R4/RConn1 -- Body4/LConn1
  R4/LConn1 -- Body3/RConn1
  Actuator4/RConn1 -- R4/LConn3
  Initi4/RConn1 -- R4/LConn2
  Sensor4/LConn1 -- R4/RConn2

== system DynTaskCon/KinematicMotionControl ==
  In1 : Inport
  Demux1 : Demux  Outputs=3
  Demux2 : Demux  Outputs=6
  Demux3 : Demux  Outputs=6
  Demux4 : Demux  Outputs=6
  Mux{1..6} (6 alike) : Mux  Inputs=3
  Out1 : Outport
  Out2 : Outport  Port=2
  Out3 : Outport  Port=3
  Out4 : Outport  Port=4
  Out5 : Outport  Port=5
  Out6 : Outport  Port=6
  wires:
  Demux1/3 -> Demux4/1
  Demux1/2 -> Demux3/1
  Demux1/1 -> Demux2/1
  Mux1/1 -> Out1/1
  Mux4/1 -> Out2/1
  Mux2/1 -> Out3/1
  In1/1 -> Demux1/1
  Mux3/1 -> Out4/1
  Mux5/1 -> Out5/1
  Mux6/1 -> Out6/1
  Demux2/1 -> Mux1/1
  Demux2/2 -> Mux4/1
  Demux2/3 -> Mux2/1
  Demux2/4 -> Mux3/1
  Demux2/5 -> Mux5/1
  Demux2/6 -> Mux6/1
  Demux3/1 -> Mux1/2
  Demux3/2 -> Mux4/2
  Demux3/3 -> Mux2/2
  Demux3/4 -> Mux3/2
  Demux3/5 -> Mux5/2
  Demux3/6 -> Mux6/2
  Demux4/1 -> Mux1/3
  Demux4/2 -> Mux4/3
  Demux4/3 -> Mux2/3
  Demux4/4 -> Mux3/3
  Demux4/5 -> Mux5/3
  Demux4/6 -> Mux6/3

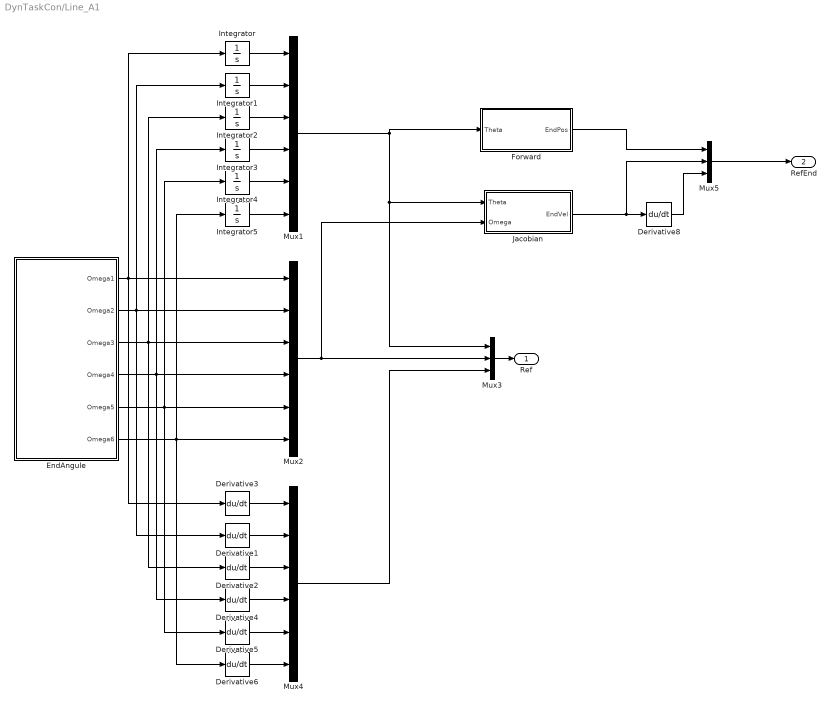
== system DynTaskCon/Line_A1 ==
  Derivative{1..6,8} (7 alike) : Derivative
  EndAngule : Subsystem
  Forward : Stateflow chart  TreatAsAtomicUnit=on
  Integrator : Integrator  InitialCondition=a1/180*pi
  Integrator1 : Integrator  InitialCondition=a2/180*pi
  Integrator2 : Integrator  InitialCondition=a3/180*pi
  Integrator3 : Integrator  InitialCondition=a4/180*pi
  Integrator4 : Integrator  InitialCondition=a5/180*pi
  Integrator5 : Integrator  InitialCondition=a6/180*pi
  Jacobian : Stateflow chart  TreatAsAtomicUnit=on
  Mux1 : Mux  Inputs=6
  Mux2 : Mux  Inputs=6
  Mux3 : Mux  Inputs=3
  Mux4 : Mux  Inputs=6
  Mux5 : Mux  Inputs=3
  Ref : Outport
  RefEnd : Outport  Port=2
  wires:
  Derivative8/1 -> Mux5/3
  Jacobian/1(EndVel) -> Derivative8/1, Mux5/2
  Forward/1(EndPos) -> Mux5/1
  Mux5/1 -> RefEnd/1
  Mux4/1 -> Mux3/3
  Mux1/1 -> Jacobian/1(Theta), Mux3/1, Forward/1(Theta)
  Mux2/1 -> Jacobian/2(Omega), Mux3/2
  Derivative6/1 -> Mux4/6
  Derivative5/1 -> Mux4/5
  Derivative4/1 -> Mux4/4
  Derivative2/1 -> Mux4/3
  Derivative1/1 -> Mux4/2
  Derivative3/1 -> Mux4/1
  Integrator5/1 -> Mux1/6
  Integrator4/1 -> Mux1/5
  Integrator3/1 -> Mux1/4
  Integrator2/1 -> Mux1/3
  Integrator1/1 -> Mux1/2
  Integrator/1 -> Mux1/1
  EndAngule/6(Omega6) -> Derivative6/1, Mux2/6, Integrator5/1
  EndAngule/5(Omega5) -> Derivative5/1, Mux2/5, Integrator4/1
  EndAngule/4(Omega4) -> Derivative4/1, Mux2/4, Integrator3/1
  EndAngule/3(Omega3) -> Derivative2/1, Mux2/3, Integrator2/1
  EndAngule/2(Omega2) -> Derivative1/1, Mux2/2, Integrator1/1
  EndAngule/1(Omega1) -> Derivative3/1, Mux2/1, Integrator/1
  Mux3/1 -> Ref/1

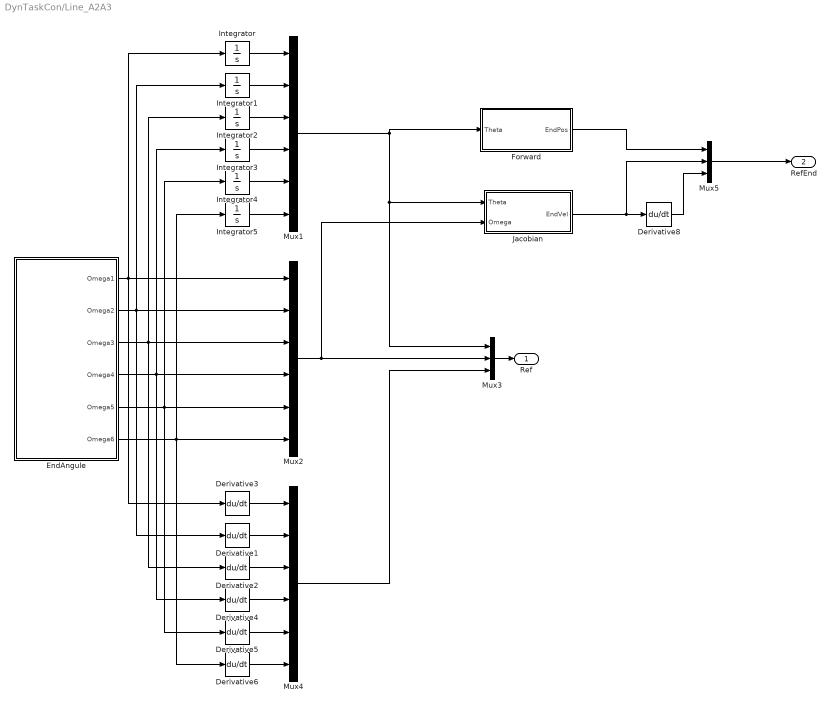
== system DynTaskCon/Line_A2A3 ==
  Derivative{1..6,8} (7 alike) : Derivative
  EndAngule : Subsystem
  Forward : Stateflow chart  TreatAsAtomicUnit=on
  Integrator : Integrator  InitialCondition=a1/180*pi
  Integrator1 : Integrator  InitialCondition=a2/180*pi
  Integrator2 : Integrator  InitialCondition=a3/180*pi
  Integrator3 : Integrator  InitialCondition=a4/180*pi
  Integrator4 : Integrator  InitialCondition=a5/180*pi
  Integrator5 : Integrator  InitialCondition=a6/180*pi
  Jacobian : Stateflow chart  TreatAsAtomicUnit=on
  Mux1 : Mux  Inputs=6
  Mux2 : Mux  Inputs=6
  Mux3 : Mux  Inputs=3
  Mux4 : Mux  Inputs=6
  Mux5 : Mux  Inputs=3
  Ref : Outport
  RefEnd : Outport  Port=2
  wires:
  Mux3/1 -> Ref/1
  EndAngule/1(Omega1) -> Integrator/1, Mux2/1, Derivative3/1
  EndAngule/2(Omega2) -> Integrator1/1, Mux2/2, Derivative1/1
  EndAngule/3(Omega3) -> Integrator2/1, Mux2/3, Derivative2/1
  EndAngule/4(Omega4) -> Integrator3/1, Mux2/4, Derivative4/1
  EndAngule/5(Omega5) -> Integrator4/1, Mux2/5, Derivative5/1
  EndAngule/6(Omega6) -> Integrator5/1, Mux2/6, Derivative6/1
  Integrator/1 -> Mux1/1
  Integrator1/1 -> Mux1/2
  Integrator2/1 -> Mux1/3
  Integrator3/1 -> Mux1/4
  Integrator4/1 -> Mux1/5
  Integrator5/1 -> Mux1/6
  Derivative3/1 -> Mux4/1
  Derivative1/1 -> Mux4/2
  Derivative2/1 -> Mux4/3
  Derivative4/1 -> Mux4/4
  Derivative5/1 -> Mux4/5
  Derivative6/1 -> Mux4/6
  Mux2/1 -> Mux3/2, Jacobian/2(Omega)
  Mux1/1 -> Forward/1(Theta), Mux3/1, Jacobian/1(Theta)
  Mux4/1 -> Mux3/3
  Mux5/1 -> RefEnd/1
  Forward/1(EndPos) -> Mux5/1
  Jacobian/1(EndVel) -> Mux5/2, Derivative8/1
  Derivative8/1 -> Mux5/3

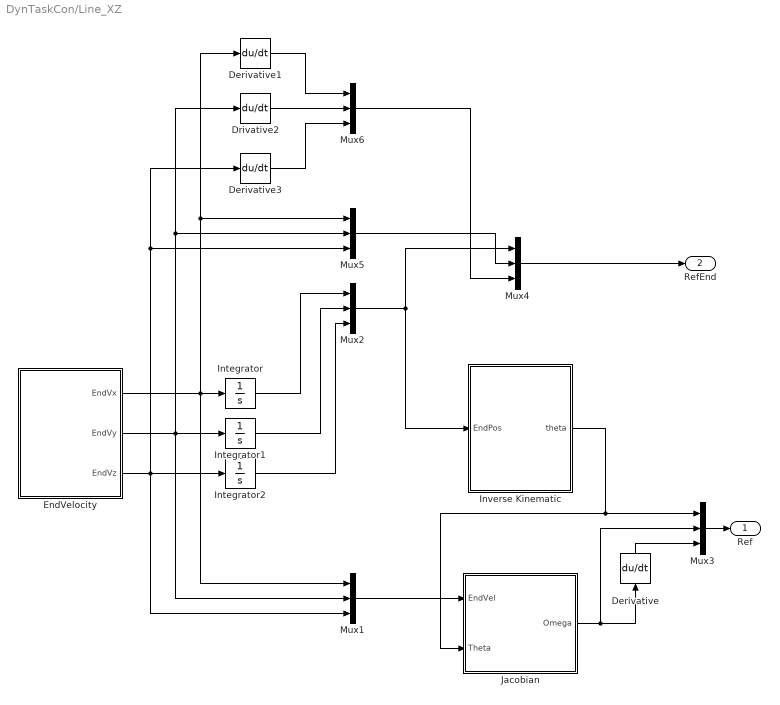
== system DynTaskCon/Line_XZ ==
  Derivative : Derivative
  Derivative1 : Derivative
  Derivative3 : Derivative
  Drivative2 : Derivative
  EndVelocity : Subsystem
  Integrator : Integrator  InitialCondition=init_Endx
  Integrator1 : Integrator  InitialCondition=init_Endy
  Integrator2 : Integrator  InitialCondition=init_Endz
  Inverse Kinematic : Stateflow chart  TreatAsAtomicUnit=on
  Jacobian : Stateflow chart  TreatAsAtomicUnit=on
  Mux{1..6} (6 alike) : Mux  Inputs=3
  Ref : Outport
  RefEnd : Outport  Port=2
  wires:
  Integrator/1 -> Mux2/1
  Integrator1/1 -> Mux2/2
  EndVelocity/1(EndVx) -> Integrator/1, Mux1/1, Mux5/1, Derivative1/1
  EndVelocity/2(EndVy) -> Integrator1/1, Mux1/2, Mux5/2, Drivative2/1
  EndVelocity/3(EndVz) -> Integrator2/1, Mux1/3, Mux5/3, Derivative3/1
  Integrator2/1 -> Mux2/3
  Mux2/1 -> Mux4/1, Inverse Kinematic/1(EndPos)
  Mux1/1 -> Jacobian/1(EndVel)
  Jacobian/1(Omega) -> Mux3/2, Derivative/1
  Mux3/1 -> Ref/1
  Derivative/1 -> Mux3/3
  Inverse Kinematic/1(theta) -> Mux3/1, Jacobian/2(Theta)
  Mux5/1 -> Mux4/2
  Mux4/1 -> RefEnd/1
  Derivative1/1 -> Mux6/1
  Drivative2/1 -> Mux6/2
  Derivative3/1 -> Mux6/3
  Mux6/1 -> Mux4/3

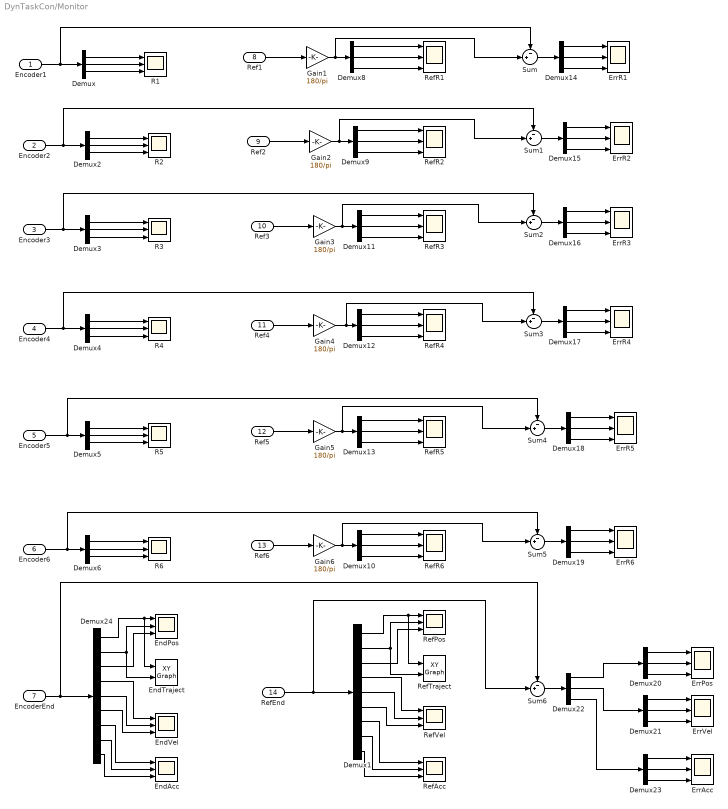
== system DynTaskCon/Monitor ==
  Encoder1 : Inport
  Encoder2 : Inport  Port=2
  Encoder3 : Inport  Port=3
  Encoder4 : Inport  Port=4
  Encoder5 : Inport  Port=5
  Encoder6 : Inport  Port=6
  EncoderEnd : Inport  Port=7
  Ref1 : Inport  Port=8
  Ref2 : Inport  Port=9
  Ref3 : Inport  Port=10
  Ref4 : Inport  Port=11
  Ref5 : Inport  Port=12
  Ref6 : Inport  Port=13
  RefEnd : Inport  Port=14
  Demux{,2..6,8..23} (22 alike) : Demux  Outputs=3
  Demux1 : Demux  Outputs=9
  Demux24 : Demux  Outputs=9
  EndAcc : Scope  NumInputPorts=3
      settings: TimeRange=0.7279693486590038  YMin=-80~-80~0.03111111111111042  YMax=60~80~0.06666666666666621  SaveName=ScopeData26
  EndPos : Scope  NumInputPorts=3
      settings: TimeRange=10  YMin=1150~-100~1518.9999998  YMax=1350~200~1519.0000003
  EndTraject : simulink/Sinks/XY Graph  SystemSampleTime=-1  xmin=1150  xmax=1350  ymin=-50  ymax=150  st=-1
  EndVel : Scope  NumInputPorts=3
      settings: YMin=-5~-5~-5  YMax=5~5~5  SaveName=ScopeData7
  ErrAcc : Scope  NumInputPorts=3
      settings: YMin=-5~-5~-5  YMax=5~5~5  SaveName=ScopeData25
  ErrPos : Scope  NumInputPorts=3
      settings: YMin=-5~-5~-5  YMax=5~5~5  SaveName=ScopeData22
  ErrR{1..6} (6 alike) : Scope  NumInputPorts=3
      ErrR1 settings: YMin=-5~-5~-5  YMax=5~5~5  SaveName=ScopeData15
      ErrR2 settings: TimeRange=10  YMin=-5~-5~-5  YMax=5~5~5  SaveName=ScopeData16
      ErrR3 settings: YMin=-5~-5~-5  YMax=5~5~5  SaveName=ScopeData17
      ErrR4 settings: YMin=-5~-5~-5  YMax=5~5~5  SaveName=ScopeData18
      ErrR5 settings: YMin=-5~-5~-5  YMax=5~5~5  SaveName=ScopeData19
      ErrR6 settings: YMin=-5~-5~-5  YMax=5~5~5  SaveName=ScopeData20
  ErrVel : Scope  NumInputPorts=3
      settings: YMin=-5~-5~-5  YMax=5~5~5  SaveName=ScopeData23
  Gain{1..6} (6 alike) : Gain  Gain=180/pi
  R{1..6} (6 alike) : Scope  NumInputPorts=3
      R1 settings: YMin=-5~-5~-5  YMax=5~5~5
      R2 settings: TimeRange=10  YMin=-1~-1~-1  YMax=1~1~1  SaveName=ScopeData2
      R3 settings: TimeRange=10  YMin=-0.35~-0.06~-0.14  YMax=0.04999999999999999~0~0.01999999999999999  SaveName=ScopeData3
      R4 settings: TimeRange=10  YMin=-1~-1~-1  YMax=1~1~1  SaveName=ScopeData4
      R5 settings: YMin=-5~-5~-5  YMax=5~5~5  SaveName=ScopeData5
      R6 settings: YMin=-5~-5~-5  YMax=5~5~5  SaveName=ScopeData6
  RefAcc : Scope  NumInputPorts=3
      settings: TimeRange=10  YMin=-5~-5~-5  YMax=5~5~5  SaveName=ScopeData24
  RefPos : Scope  NumInputPorts=3
      settings: YMin=-5~-5~-5  YMax=5~5~5  SaveName=ScopeData8
  RefR{1..6} (6 alike) : Scope  NumInputPorts=3
      RefR1 settings: YMin=-5~-5~-5  YMax=5~5~5  SaveName=ScopeData9
      RefR2 settings: YMin=-5~-5~-5  YMax=5~5~5  SaveName=ScopeData10
      RefR3 settings: YMin=-5~-5~-5  YMax=5~5~5  SaveName=ScopeData11
      RefR4 settings: YMin=-5~-5~-5  YMax=5~5~5  SaveName=ScopeData12
      RefR5 settings: YMin=-5~-5~-5  YMax=5~5~5  SaveName=ScopeData13
      RefR6 settings: YMin=-5~-5~-5  YMax=5~5~5  SaveName=ScopeData14
  RefTraject : simulink/Sinks/XY Graph  SystemSampleTime=-1  xmin=1150  xmax=1350  ymin=-50  ymax=150  st=-1
  RefVel : Scope  NumInputPorts=3
      settings: TimeRange=10  YMin=0~-1~-1  YMax=60~1~1  SaveName=ScopeData21
  Sum{,1..6} (7 alike) : Sum  Inputs=-+|
  wires:
  Demux/1 -> R1/1
  Demux/2 -> R1/2
  Demux/3 -> R1/3
  Demux2/2 -> R2/2
  Demux2/3 -> R2/3
  Demux3/2 -> R3/2
  Demux3/3 -> R3/3
  Demux4/2 -> R4/2
  Demux4/3 -> R4/3
  Demux2/1 -> R2/1
  Demux4/1 -> R4/1
  Demux3/1 -> R3/1
  Demux5/2 -> R5/2
  Demux5/3 -> R5/3
  Demux6/2 -> R6/2
  Demux6/3 -> R6/3
  Demux5/1 -> R5/1
  Demux6/1 -> R6/1
  Encoder1/1 -> Demux/1, Sum/1
  Encoder2/1 -> Demux2/1, Sum1/1
  Encoder3/1 -> Demux3/1, Sum2/1
  Encoder4/1 -> Demux4/1, Sum3/1
  Encoder5/1 -> Demux5/1, Sum4/1
  Encoder6/1 -> Demux6/1, Sum5/1
  Gain1/1 -> Demux8/1, Sum/2
  Demux8/1 -> RefR1/1
  Demux8/2 -> RefR1/2
  Demux8/3 -> RefR1/3
  Gain2/1 -> Demux9/1, Sum1/2
  Demux9/1 -> RefR2/1
  Demux9/2 -> RefR2/2
  Demux9/3 -> RefR2/3
  Gain3/1 -> Demux11/1, Sum2/2
  Demux11/1 -> RefR3/1
  Demux11/2 -> RefR3/2
  Demux11/3 -> RefR3/3
  Gain4/1 -> Demux12/1, Sum3/2
  Demux12/1 -> RefR4/1
  Demux12/2 -> RefR4/2
  Demux12/3 -> RefR4/3
  Gain5/1 -> Demux13/1, Sum4/2
  Demux13/1 -> RefR5/1
  Demux13/2 -> RefR5/2
  Demux13/3 -> RefR5/3
  Gain6/1 -> Demux10/1, Sum5/2
  Demux10/1 -> RefR6/1
  Demux10/2 -> RefR6/2
  Demux10/3 -> RefR6/3
  Ref1/1 -> Gain1/1
  Ref2/1 -> Gain2/1
  Ref3/1 -> Gain3/1
  Ref6/1 -> Gain6/1
  Ref5/1 -> Gain5/1
  Ref4/1 -> Gain4/1
  Sum/1 -> Demux14/1
  Demux14/1 -> ErrR1/1
  Demux14/2 -> ErrR1/2
  Demux14/3 -> ErrR1/3
  Sum1/1 -> Demux15/1
  Demux15/1 -> ErrR2/1
  Demux15/2 -> ErrR2/2
  Demux15/3 -> ErrR2/3
  Sum2/1 -> Demux16/1
  Demux16/1 -> ErrR3/1
  Demux16/2 -> ErrR3/2
  Demux16/3 -> ErrR3/3
  Sum3/1 -> Demux17/1
  Demux17/1 -> ErrR4/1
  Demux17/2 -> ErrR4/2
  Demux17/3 -> ErrR4/3
  Sum4/1 -> Demux18/1
  Demux18/1 -> ErrR5/1
  Demux18/2 -> ErrR5/2
  Demux18/3 -> ErrR5/3
  Sum5/1 -> Demux19/1
  Demux19/1 -> ErrR6/1
  Demux19/2 -> ErrR6/2
  Demux19/3 -> ErrR6/3
  EncoderEnd/1 -> Sum6/1, Demux24/1
  RefEnd/1 -> Sum6/2, Demux1/1
  Demux20/1 -> ErrPos/1
  Demux20/2 -> ErrPos/2
  Demux20/3 -> ErrPos/3
  Sum6/1 -> Demux22/1
  Demux22/1 -> Demux20/1
  Demux22/2 -> Demux21/1
  Demux21/1 -> ErrVel/1
  Demux21/2 -> ErrVel/2
  Demux21/3 -> ErrVel/3
  Demux1/1 -> RefPos/1, RefTraject/1
  Demux1/2 -> RefPos/2, RefTraject/2
  Demux1/3 -> RefPos/3
  Demux1/4 -> RefVel/1
  Demux1/5 -> RefVel/2
  Demux1/6 -> RefVel/3
  Demux1/7 -> RefAcc/1
  Demux1/8 -> RefAcc/2
  Demux1/9 -> RefAcc/3
  Demux23/1 -> ErrAcc/1
  Demux23/2 -> ErrAcc/2
  Demux23/3 -> ErrAcc/3
  Demux22/3 -> Demux23/1
  Demux24/1 -> EndPos/1, EndTraject/1
  Demux24/2 -> EndPos/2, EndTraject/2
  Demux24/3 -> EndPos/3
  Demux24/4 -> EndVel/1
  Demux24/5 -> EndVel/2
  Demux24/6 -> EndVel/3
  Demux24/7 -> EndAcc/1
  Demux24/8 -> EndAcc/2
  Demux24/9 -> EndAcc/3

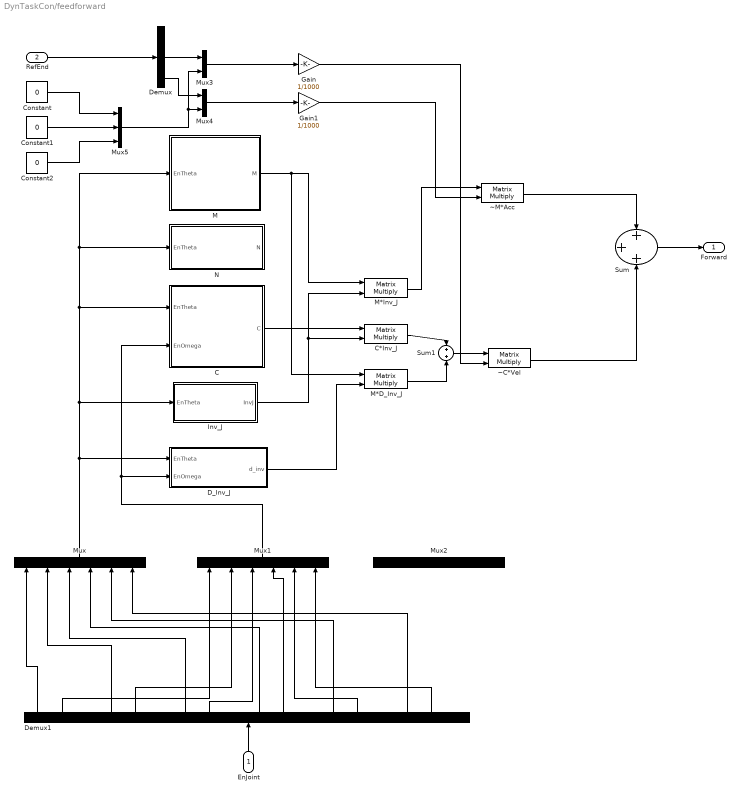
== system DynTaskCon/feedforward ==
  EnJoint : Inport
  RefEnd : Inport  Port=2
  C : Stateflow chart  TreatAsAtomicUnit=on
  C*Inv_J : Product  Multiplication=Matrix(*)  RndMeth=Zero
  Constant : Constant  Value=0
  Constant1 : Constant  Value=0
  Constant2 : Constant  Value=0
  D_Inv_J : Stateflow chart  TreatAsAtomicUnit=on
  Demux : Demux  Outputs=3
  Demux1 : Demux  Outputs=18
  Gain : Gain  Gain=1/1000
  Gain1 : Gain  Gain=1/1000
  Inv_J : Stateflow chart  TreatAsAtomicUnit=on
  M : Stateflow chart  TreatAsAtomicUnit=on
  M*D_Inv_J : Product  Multiplication=Matrix(*)  RndMeth=Zero
  M*Inv_J : Product  Multiplication=Matrix(*)  RndMeth=Zero
  Mux : Mux  Inputs=6
  Mux1 : Mux  Inputs=6
  Mux2 : Mux  Inputs=6
  Mux3 : Mux  Inputs=2
  Mux4 : Mux  Inputs=2
  Mux5 : Mux  Inputs=3
  N : Stateflow chart  TreatAsAtomicUnit=on
  Sum : Sum  Inputs=+++
  Sum1 : Sum  Inputs=+|+
  ~C*Vel : Product  Multiplication=Matrix(*)  RndMeth=Zero
  ~M*Acc : Product  Multiplication=Matrix(*)  RndMeth=Zero
  Forward : Outport
  wires:
  Sum/1 -> Forward/1
  EnJoint/1 -> Demux1/1
  Mux/1 -> M/1(EnTheta), N/1(EnTheta), C/1(EnTheta), Inv_J/1(EnTheta), D_Inv_J/1(EnTheta)
  Mux1/1 -> C/2(EnOmega), D_Inv_J/2(EnOmega)
  RefEnd/1 -> Demux/1
  Demux/2 -> Mux3/1
  M/1(M) -> M*Inv_J/1, M*D_Inv_J/1
  Inv_J/1(InvJ) -> M*Inv_J/2, C*Inv_J/2
  C/1(C) -> C*Inv_J/1
  D_Inv_J/1(d_inv) -> M*D_Inv_J/2
  C*Inv_J/1 -> Sum1/1
  M*D_Inv_J/1 -> Sum1/2
  M*Inv_J/1 -> ~M*Acc/1
  Mux4/1 -> Gain1/1
  Sum1/1 -> ~C*Vel/1
  Mux3/1 -> Gain/1
  ~M*Acc/1 -> Sum/1
  ~C*Vel/1 -> Sum/3
  Demux/3 -> Mux4/1
  Constant/1 -> Mux5/1
  Constant1/1 -> Mux5/2
  Constant2/1 -> Mux5/3
  Mux5/1 -> Mux3/2, Mux4/2
  Gain/1 -> ~C*Vel/2
  Gain1/1 -> ~M*Acc/2
  Demux1/1 -> Mux/1
  Demux1/4 -> Mux/2
  Demux1/7 -> Mux/3
  Demux1/10 -> Mux/4
  Demux1/13 -> Mux/5
  Demux1/16 -> Mux/6
  Demux1/2 -> Mux1/1
  Demux1/5 -> Mux1/2
  Demux1/8 -> Mux1/3
  Demux1/11 -> Mux1/4
  Demux1/14 -> Mux1/5
  Demux1/17 -> Mux1/6

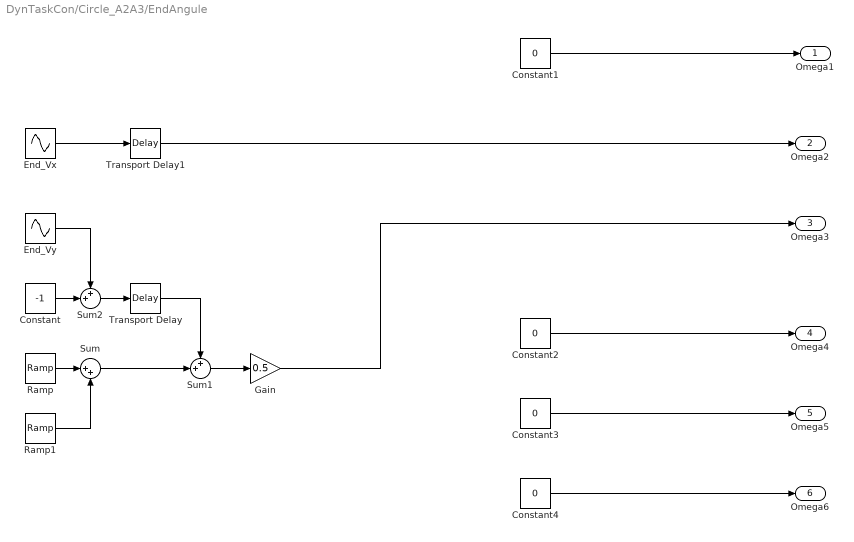
== system DynTaskCon/Circle_A2A3/EndAngule ==
  Constant : Constant  Value=-1
  Constant{1..4} (4 alike) : Constant  Value=0
  End_Vx : Sin  Amplitude=0.5  Frequency=freq  SampleTime=0
  End_Vy : Sin  Frequency=freq  Phase=pi/2  SampleTime=0
  Gain : Gain  Gain=0.5
  Ramp : simulink/Sources/Ramp  SystemSampleTime=-1  slope=1  start=0  X0=0
  Ramp1 : simulink/Sources/Ramp  SystemSampleTime=-1  slope=-1  start=1  X0=0
  Sum : Sum  Inputs=|++
  Sum1 : Sum  Inputs=++|
  Sum2 : Sum  Inputs=++|
  Transport Delay : TransportDelay
  Transport Delay1 : TransportDelay
  Omega1 : Outport
  Omega2 : Outport  Port=2
  Omega3 : Outport  Port=3
  Omega4 : Outport  Port=4
  Omega5 : Outport  Port=5
  Omega6 : Outport  Port=6
  wires:
  Constant1/1 -> Omega1/1
  Constant3/1 -> Omega5/1
  Constant4/1 -> Omega6/1
  Constant2/1 -> Omega4/1
  End_Vy/1 -> Sum2/1
  Ramp/1 -> Sum/1
  Ramp1/1 -> Sum/2
  Transport Delay/1 -> Sum1/1
  Sum2/1 -> Transport Delay/1
  Constant/1 -> Sum2/2
  Sum/1 -> Sum1/2
  Sum1/1 -> Gain/1
  End_Vx/1 -> Transport Delay1/1
  Transport Delay1/1 -> Omega2/1
  Gain/1 -> Omega3/1

== system DynTaskCon/Circle_XY/EndVelocity ==
  Constant : Constant  Value=-1
  End_Vx : Sin  Amplitude=-tvel  Frequency=freq  SampleTime=0
  End_Vy : Sin  Frequency=freq  Phase=pi/2  SampleTime=0
  End_Vz : Constant  Value=0
  Gain : Gain  Gain=tvel
  Ramp : simulink/Sources/Ramp  SystemSampleTime=-1  slope=1  start=0  X0=0
  Ramp1 : simulink/Sources/Ramp  SystemSampleTime=-1  slope=-1  start=1  X0=0
  Sum : Sum  Inputs=|++
  Sum1 : Sum  Inputs=++|
  Sum2 : Sum  Inputs=++|
  Transport Delay : TransportDelay
  Transport Delay1 : TransportDelay
  EndVx : Outport
  EndVy : Outport  Port=2
  EndVz : Outport  Port=3
  wires:
  End_Vy/1 -> Sum2/1
  Ramp/1 -> Sum/1
  Ramp1/1 -> Sum/2
  Transport Delay/1 -> Sum1/1
  Sum2/1 -> Transport Delay/1
  Constant/1 -> Sum2/2
  Sum/1 -> Sum1/2
  Sum1/1 -> Gain/1
  End_Vx/1 -> Transport Delay1/1
  Gain/1 -> EndVy/1
  End_Vz/1 -> EndVz/1
  Transport Delay1/1 -> EndVx/1

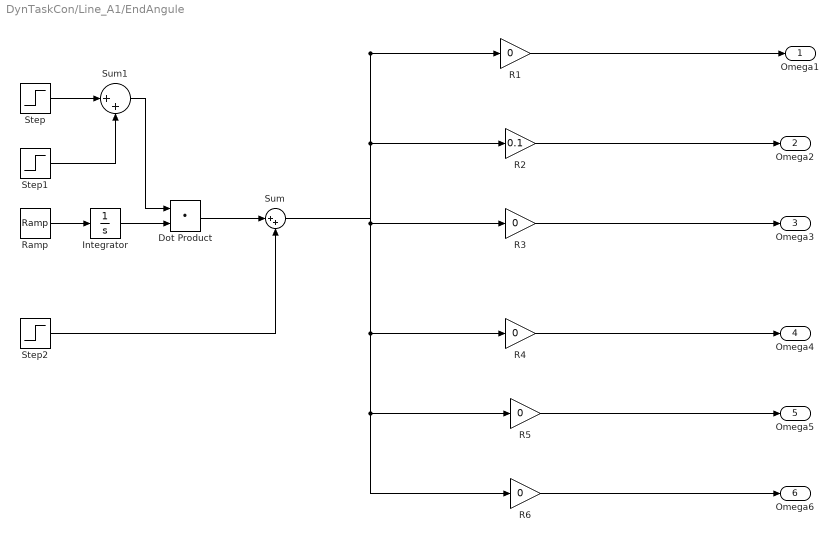
== system DynTaskCon/Line_A1/EndAngule ==
  Dot Product : DotProduct  InputSameDT=on  OutDataTypeStr=Inherit: Inherit via internal rule
  Integrator : Integrator
  R{1,3..6} (5 alike) : Gain  Gain=0
  R2 : Gain  Gain=0.1
  Ramp : simulink/Sources/Ramp  SystemSampleTime=-1  slope=1  start=0  X0=0
  Step : Step  After=-2  SampleTime=0
  Step1 : Step  Time=0  After=2  SampleTime=0
  Step2 : Step  SampleTime=0
  Sum : Sum  Inputs=|++
  Sum1 : Sum  Inputs=|++
  Omega1 : Outport
  Omega2 : Outport  Port=2
  Omega3 : Outport  Port=3
  Omega4 : Outport  Port=4
  Omega5 : Outport  Port=5
  Omega6 : Outport  Port=6
  wires:
  R4/1 -> Omega4/1
  R6/1 -> Omega6/1
  R5/1 -> Omega5/1
  R3/1 -> Omega3/1
  R2/1 -> Omega2/1
  Ramp/1 -> Integrator/1
  R1/1 -> Omega1/1
  Sum/1 -> R1/1, R2/1, R3/1, R4/1, R5/1, R6/1
  Integrator/1 -> Dot Product/2
  Step/1 -> Sum1/1
  Sum1/1 -> Dot Product/1
  Dot Product/1 -> Sum/1
  Step2/1 -> Sum/2
  Step1/1 -> Sum1/2

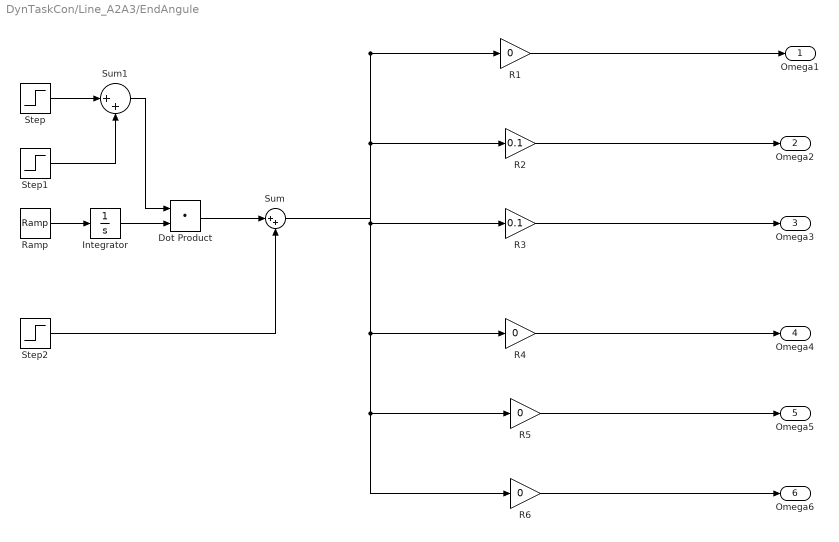
== system DynTaskCon/Line_A2A3/EndAngule ==
  Dot Product : DotProduct  InputSameDT=on  OutDataTypeStr=Inherit: Inherit via internal rule
  Integrator : Integrator
  R{1,4..6} (4 alike) : Gain  Gain=0
  R2 : Gain  Gain=0.1
  R3 : Gain  Gain=0.1
  Ramp : simulink/Sources/Ramp  SystemSampleTime=-1  slope=1  start=0  X0=0
  Step : Step  After=-2  SampleTime=0
  Step1 : Step  Time=0  After=2  SampleTime=0
  Step2 : Step  SampleTime=0
  Sum : Sum  Inputs=|++
  Sum1 : Sum  Inputs=|++
  Omega1 : Outport
  Omega2 : Outport  Port=2
  Omega3 : Outport  Port=3
  Omega4 : Outport  Port=4
  Omega5 : Outport  Port=5
  Omega6 : Outport  Port=6
  wires:
  Step1/1 -> Sum1/2
  Step2/1 -> Sum/2
  Dot Product/1 -> Sum/1
  Sum1/1 -> Dot Product/1
  Step/1 -> Sum1/1
  Integrator/1 -> Dot Product/2
  Sum/1 -> R6/1, R5/1, R4/1, R3/1, R2/1, R1/1
  R1/1 -> Omega1/1
  Ramp/1 -> Integrator/1
  R2/1 -> Omega2/1
  R3/1 -> Omega3/1
  R5/1 -> Omega5/1
  R6/1 -> Omega6/1
  R4/1 -> Omega4/1

== system DynTaskCon/Line_XZ/EndVelocity ==
  Dot Product : DotProduct  InputSameDT=on  OutDataTypeStr=Inherit: Inherit via internal rule
  Gain : Gain  Gain=30
  Gain1 : Gain  Gain=0
  Gain2 : Gain  Gain=30
  Integrator : Integrator
  Ramp : simulink/Sources/Ramp  SystemSampleTime=-1  slope=1  start=0  X0=0
  Step : Step  After=-2  SampleTime=0
  Step1 : Step  Time=0  After=2  SampleTime=0
  Step2 : Step  SampleTime=0
  Sum : Sum  Inputs=|++
  Sum1 : Sum  Inputs=|++
  EndVx : Outport
  EndVy : Outport  Port=2
  EndVz : Outport  Port=3
  wires:
  Step1/1 -> Sum1/2
  Step2/1 -> Sum/2
  Dot Product/1 -> Sum/1
  Sum1/1 -> Dot Product/1
  Step/1 -> Sum1/1
  Integrator/1 -> Dot Product/2
  Ramp/1 -> Integrator/1
  Gain/1 -> EndVx/1
  Gain1/1 -> EndVy/1
  Gain2/1 -> EndVz/1
  Sum/1 -> Gain/1, Gain1/1, Gain2/1

== matlab function Circle_XY/Jacobian ==
  data: Omega output double; EndVel input double; Theta input double; L parameter double
function Omega = fcn(EndVel,Theta,L)
%#eml

Omega = zeros(6,1);
V = [EndVel; 0; 0; 0];   
g = fwd_kin(L,Theta');
Jb = body_Jacobian(L,Theta');
Adg_inv = double(AdjointInv(g));
Omega = double((Jb \ Adg_inv* V)')';

== matlab function Circle_XY/Inverse Kinematic ==
  data: EndPos input double; init_Rot parameter double; theta output double; L parameter double
function theta = fcn(EndPos,init_Rot,L)
%#eml
theta =[0;0; 0; 0; 0; 0];
gd = [init_Rot,EndPos;[0 0 0],1];
[theta_total,num_total] = inv_kin(gd,L);
theta = theta_total(:,2);

== matlab function feedforward/D_Inv_J ==
  data: EnTheta input double; d_inv output double; EnOmega input double; L parameter double
function d_inv = fcn(EnTheta,EnOmega,L)
%#eml
L = L/1000;
d_inv = zeros(6);
d_inv = d_inv + d_inv_SJ_1(L,EnTheta')*EnOmega(1);
d_inv = d_inv + d_inv_SJ_2(L,EnTheta')*EnOmega(2);
d_inv = d_inv + d_inv_SJ_3(L,EnTheta')*EnOmega(3);
d_inv = d_inv + d_inv_SJ_4(L,EnTheta')*EnOmega(4);
d_inv = d_inv + d_inv_SJ_5(L,EnTheta')*EnOmega(5);
d_inv = d_inv + d_inv_SJ_6(L,EnTheta')*EnOmega(6);
